simulink model "HybridFEMModel"  (Simulink 7.0)
settings: Solver=FixedStepDiscrete  SolverMode=SingleTasking  StartTime=0.0  StopTime=RunningTime  FixedStep=SampleRate  RelTol=1e-3
undefined symbols (not defined in the file): Alpham, DiscIntNeverNeededParam, Elements, gamma1, gamma2, sample, SampleRate
libraries: simulink x8
(part 2 of 2)

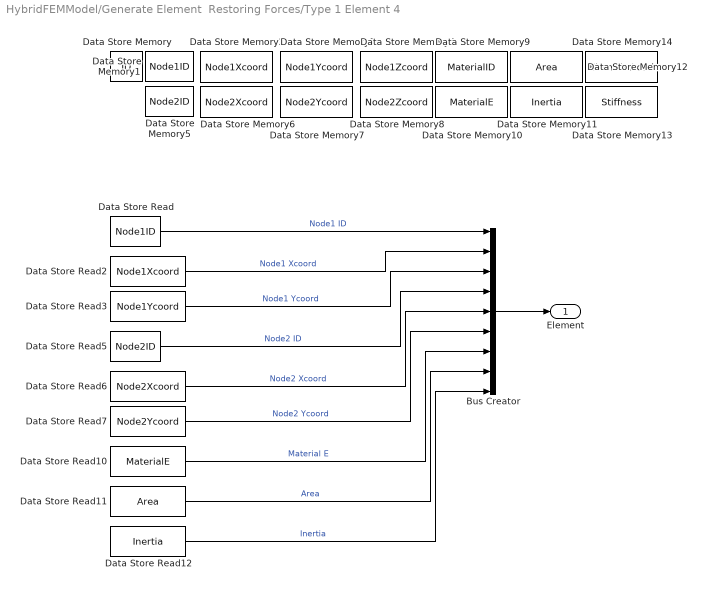
== system HybridFEMModel/Generate Element  Restoring Forces/Type 1 Element 4 ==
  Bus Creator : BusCreator  Inputs=9
  Data Store Memory : DataStoreMemory  DataStoreName=ID  InitialValue=Elements(id).ID  OutDataType=sfix(16)  OutScaling=2^0
  Data Store Memory1 : DataStoreMemory  DataStoreName=Node1ID  InitialValue=Elements(id).Nodes(1).ID  OutDataType=sfix(16)  OutScaling=2^0
  Data Store Memory10 : DataStoreMemory  DataStoreName=MaterialE  InitialValue=Elements(id).Material(1).E  OutDataType=sfix(16)  OutScaling=2^0
  Data Store Memory11 : DataStoreMemory  DataStoreName=Inertia  InitialValue=Elements(id).Inertia  OutDataType=sfix(16)  OutScaling=2^0
  Data Store Memory12 : DataStoreMemory  DataStoreName=Area  InitialValue=Elements(id).Area  OutDataType=sfix(16)  OutScaling=2^0
  Data Store Memory13 : DataStoreMemory  DataStoreName=Stiffness  InitialValue=Elements(id).Stiffness  OutDataType=sfix(16)  OutScaling=2^0
  Data Store Memory14 : DataStoreMemory  DataStoreName=ElemDistLoad  InitialValue=Elements(id).ElemDistLoad  OutDataType=sfix(16)  OutScaling=2^0
  Data Store Memory2 : DataStoreMemory  DataStoreName=Node1Xcoord  InitialValue=Elements(id).Nodes(1).Xcoord  OutDataType=sfix(16)  OutScaling=2^0
  Data Store Memory3 : DataStoreMemory  DataStoreName=Node1Ycoord  InitialValue=Elements(id).Nodes(1).Ycoord  OutDataType=sfix(16)  OutScaling=2^0
  Data Store Memory4 : DataStoreMemory  DataStoreName=Node1Zcoord  InitialValue=Elements(id).Nodes(1).Zcoord  OutDataType=sfix(16)  OutScaling=2^0
  Data Store Memory5 : DataStoreMemory  DataStoreName=Node2ID  InitialValue=Elements(id).Nodes(2).ID  OutDataType=sfix(16)  OutScaling=2^0
  Data Store Memory6 : DataStoreMemory  DataStoreName=Node2Xcoord  InitialValue=Elements(id).Nodes(2).Xcoord  OutDataType=sfix(16)  OutScaling=2^0
  Data Store Memory7 : DataStoreMemory  DataStoreName=Node2Ycoord  InitialValue=Elements(id).Nodes(2).Ycoord  OutDataType=sfix(16)  OutScaling=2^0
  Data Store Memory8 : DataStoreMemory  DataStoreName=Node2Zcoord  InitialValue=Elements(id).Nodes(2).Zcoord  OutDataType=sfix(16)  OutScaling=2^0
  Data Store Memory9 : DataStoreMemory  DataStoreName=MaterialID  InitialValue=Elements(id).Material(1).ID  OutDataType=sfix(16)  OutScaling=2^0
  Data Store Read : DataStoreRead  DataStoreName=Node1ID  SampleTime=-1
  Data Store Read10 : DataStoreRead  DataStoreName=MaterialE  SampleTime=-1
  Data Store Read11 : DataStoreRead  DataStoreName=Area  SampleTime=-1
  Data Store Read12 : DataStoreRead  DataStoreName=Inertia  SampleTime=-1
  Data Store Read2 : DataStoreRead  DataStoreName=Node1Xcoord  SampleTime=-1
  Data Store Read3 : DataStoreRead  DataStoreName=Node1Ycoord  SampleTime=-1
  Data Store Read5 : DataStoreRead  DataStoreName=Node2ID  SampleTime=-1
  Data Store Read6 : DataStoreRead  DataStoreName=Node2Xcoord  SampleTime=-1
  Data Store Read7 : DataStoreRead  DataStoreName=Node2Ycoord  SampleTime=-1
  Element : Outport  OutDataType=sfix(16)  OutScaling=2^0
  wires:
  Bus Creator/1 -> Element/1
  Data Store Read/1 -> Bus Creator/1  "Node1 ID"
  Data Store Read2/1 -> Bus Creator/2  "Node1 Xcoord"
  Data Store Read3/1 -> Bus Creator/3  "Node1 Ycoord"
  Data Store Read5/1 -> Bus Creator/4  "Node2 ID"
  Data Store Read6/1 -> Bus Creator/5  "Node2 Xcoord"
  Data Store Read7/1 -> Bus Creator/6  "Node2 Ycoord"
  Data Store Read10/1 -> Bus Creator/7  "Material E"
  Data Store Read11/1 -> Bus Creator/8  "Area"
  Data Store Read12/1 -> Bus Creator/9  "Inertia"

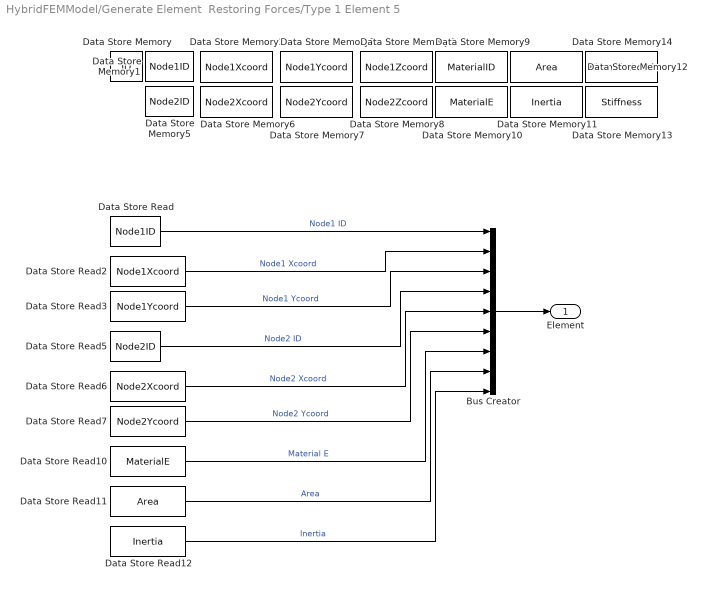
== system HybridFEMModel/Generate Element  Restoring Forces/Type 1 Element 5 ==
  Bus Creator : BusCreator  Inputs=9
  Data Store Memory : DataStoreMemory  DataStoreName=ID  InitialValue=Elements(id).ID  OutDataType=sfix(16)  OutScaling=2^0
  Data Store Memory1 : DataStoreMemory  DataStoreName=Node1ID  InitialValue=Elements(id).Nodes(1).ID  OutDataType=sfix(16)  OutScaling=2^0
  Data Store Memory10 : DataStoreMemory  DataStoreName=MaterialE  InitialValue=Elements(id).Material(1).E  OutDataType=sfix(16)  OutScaling=2^0
  Data Store Memory11 : DataStoreMemory  DataStoreName=Inertia  InitialValue=Elements(id).Inertia  OutDataType=sfix(16)  OutScaling=2^0
  Data Store Memory12 : DataStoreMemory  DataStoreName=Area  InitialValue=Elements(id).Area  OutDataType=sfix(16)  OutScaling=2^0
  Data Store Memory13 : DataStoreMemory  DataStoreName=Stiffness  InitialValue=Elements(id).Stiffness  OutDataType=sfix(16)  OutScaling=2^0
  Data Store Memory14 : DataStoreMemory  DataStoreName=ElemDistLoad  InitialValue=Elements(id).ElemDistLoad  OutDataType=sfix(16)  OutScaling=2^0
  Data Store Memory2 : DataStoreMemory  DataStoreName=Node1Xcoord  InitialValue=Elements(id).Nodes(1).Xcoord  OutDataType=sfix(16)  OutScaling=2^0
  Data Store Memory3 : DataStoreMemory  DataStoreName=Node1Ycoord  InitialValue=Elements(id).Nodes(1).Ycoord  OutDataType=sfix(16)  OutScaling=2^0
  Data Store Memory4 : DataStoreMemory  DataStoreName=Node1Zcoord  InitialValue=Elements(id).Nodes(1).Zcoord  OutDataType=sfix(16)  OutScaling=2^0
  Data Store Memory5 : DataStoreMemory  DataStoreName=Node2ID  InitialValue=Elements(id).Nodes(2).ID  OutDataType=sfix(16)  OutScaling=2^0
  Data Store Memory6 : DataStoreMemory  DataStoreName=Node2Xcoord  InitialValue=Elements(id).Nodes(2).Xcoord  OutDataType=sfix(16)  OutScaling=2^0
  Data Store Memory7 : DataStoreMemory  DataStoreName=Node2Ycoord  InitialValue=Elements(id).Nodes(2).Ycoord  OutDataType=sfix(16)  OutScaling=2^0
  Data Store Memory8 : DataStoreMemory  DataStoreName=Node2Zcoord  InitialValue=Elements(id).Nodes(2).Zcoord  OutDataType=sfix(16)  OutScaling=2^0
  Data Store Memory9 : DataStoreMemory  DataStoreName=MaterialID  InitialValue=Elements(id).Material(1).ID  OutDataType=sfix(16)  OutScaling=2^0
  Data Store Read : DataStoreRead  DataStoreName=Node1ID  SampleTime=-1
  Data Store Read10 : DataStoreRead  DataStoreName=MaterialE  SampleTime=-1
  Data Store Read11 : DataStoreRead  DataStoreName=Area  SampleTime=-1
  Data Store Read12 : DataStoreRead  DataStoreName=Inertia  SampleTime=-1
  Data Store Read2 : DataStoreRead  DataStoreName=Node1Xcoord  SampleTime=-1
  Data Store Read3 : DataStoreRead  DataStoreName=Node1Ycoord  SampleTime=-1
  Data Store Read5 : DataStoreRead  DataStoreName=Node2ID  SampleTime=-1
  Data Store Read6 : DataStoreRead  DataStoreName=Node2Xcoord  SampleTime=-1
  Data Store Read7 : DataStoreRead  DataStoreName=Node2Ycoord  SampleTime=-1
  Element : Outport  OutDataType=sfix(16)  OutScaling=2^0
  wires:
  Data Store Read12/1 -> Bus Creator/9  "Inertia"
  Data Store Read11/1 -> Bus Creator/8  "Area"
  Data Store Read10/1 -> Bus Creator/7  "Material E"
  Data Store Read7/1 -> Bus Creator/6  "Node2 Ycoord"
  Data Store Read6/1 -> Bus Creator/5  "Node2 Xcoord"
  Data Store Read5/1 -> Bus Creator/4  "Node2 ID"
  Data Store Read3/1 -> Bus Creator/3  "Node1 Ycoord"
  Data Store Read2/1 -> Bus Creator/2  "Node1 Xcoord"
  Data Store Read/1 -> Bus Creator/1  "Node1 ID"
  Bus Creator/1 -> Element/1

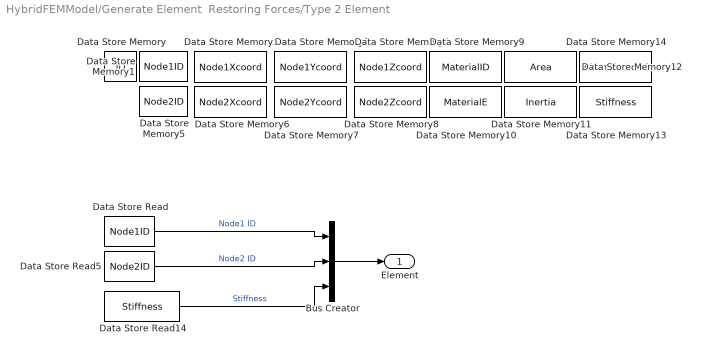
== system HybridFEMModel/Generate Element  Restoring Forces/Type 2 Element ==
  Bus Creator : BusCreator  Inputs=3
  Data Store Memory : DataStoreMemory  DataStoreName=ID  InitialValue=Elements(id).ID  OutDataType=sfix(16)  OutScaling=2^0
  Data Store Memory1 : DataStoreMemory  DataStoreName=Node1ID  InitialValue=Elements(id).Nodes(1).ID  OutDataType=sfix(16)  OutScaling=2^0
  Data Store Memory10 : DataStoreMemory  DataStoreName=MaterialE  InitialValue=Elements(id).Material(1).E  OutDataType=sfix(16)  OutScaling=2^0
  Data Store Memory11 : DataStoreMemory  DataStoreName=Inertia  InitialValue=Elements(id).Inertia  OutDataType=sfix(16)  OutScaling=2^0
  Data Store Memory12 : DataStoreMemory  DataStoreName=Area  InitialValue=Elements(id).Area  OutDataType=sfix(16)  OutScaling=2^0
  Data Store Memory13 : DataStoreMemory  DataStoreName=Stiffness  InitialValue=Elements(id).Stiffness  OutDataType=sfix(16)  OutScaling=2^0
  Data Store Memory14 : DataStoreMemory  DataStoreName=ElemDistLoad  InitialValue=Elements(id).ElemDistLoad  OutDataType=sfix(16)  OutScaling=2^0
  Data Store Memory2 : DataStoreMemory  DataStoreName=Node1Xcoord  InitialValue=Elements(id).Nodes(1).Xcoord  OutDataType=sfix(16)  OutScaling=2^0
  Data Store Memory3 : DataStoreMemory  DataStoreName=Node1Ycoord  InitialValue=Elements(id).Nodes(1).Ycoord  OutDataType=sfix(16)  OutScaling=2^0
  Data Store Memory4 : DataStoreMemory  DataStoreName=Node1Zcoord  InitialValue=Elements(id).Nodes(1).Zcoord  OutDataType=sfix(16)  OutScaling=2^0
  Data Store Memory5 : DataStoreMemory  DataStoreName=Node2ID  InitialValue=Elements(id).Nodes(2).ID  OutDataType=sfix(16)  OutScaling=2^0
  Data Store Memory6 : DataStoreMemory  DataStoreName=Node2Xcoord  InitialValue=Elements(id).Nodes(2).Xcoord  OutDataType=sfix(16)  OutScaling=2^0
  Data Store Memory7 : DataStoreMemory  DataStoreName=Node2Ycoord  InitialValue=Elements(id).Nodes(2).Ycoord  OutDataType=sfix(16)  OutScaling=2^0
  Data Store Memory8 : DataStoreMemory  DataStoreName=Node2Zcoord  InitialValue=Elements(id).Nodes(2).Zcoord  OutDataType=sfix(16)  OutScaling=2^0
  Data Store Memory9 : DataStoreMemory  DataStoreName=MaterialID  InitialValue=Elements(id).Material(1).ID  OutDataType=sfix(16)  OutScaling=2^0
  Data Store Read : DataStoreRead  DataStoreName=Node1ID  SampleTime=-1
  Data Store Read14 : DataStoreRead  DataStoreName=Stiffness  SampleTime=-1
  Data Store Read5 : DataStoreRead  DataStoreName=Node2ID  SampleTime=-1
  Element : Outport  OutDataType=sfix(16)  OutScaling=2^0
  wires:
  Data Store Read14/1 -> Bus Creator/3  "Stiffness"
  Data Store Read5/1 -> Bus Creator/2  "Node2 ID"
  Data Store Read/1 -> Bus Creator/1  "Node1 ID"
  Bus Creator/1 -> Element/1

== system HybridFEMModel/Generate Element  Restoring Forces1/Generate Type 2 Element Restoring Force ==
  Displacement : Inport  OutDataType=sfix(16)  OutScaling=2^0
  Velocity : Inport  Port=2  OutDataType=sfix(16)  OutScaling=2^0
  Element : Inport  Port=3  OutDataType=sfix(16)  OutScaling=2^0
  Timestep : Inport  Port=4  OutDataType=sfix(16)  OutScaling=2^0
  Generate Actuator Command : Stateflow chart
  Act Cmd (m) : Outport  OutDataType=sfix(16)  OutScaling=2^0
  QuadRampCoeffs : Outport  Port=2  OutDataType=sfix(16)  OutScaling=2^0
  wires:
  Generate Actuator Command/1(Command) -> Act Cmd (m)/1
  Displacement/1 -> Generate Actuator Command/2(Displacement)
  Element/1 -> Generate Actuator Command/1(Element)
  Velocity/1 -> Generate Actuator Command/3(Velocity)
  Timestep/1 -> Generate Actuator Command/4(Timestep)
  Generate Actuator Command/2(QuadRampCoeffs) -> QuadRampCoeffs/1

== system HybridFEMModel/Generate Element  Restoring Forces1/Type 2 Element ==
  Bus Creator : BusCreator  Inputs=3
  Data Store Memory : DataStoreMemory  DataStoreName=ID  InitialValue=Elements(id).ID  OutDataType=sfix(16)  OutScaling=2^0
  Data Store Memory1 : DataStoreMemory  DataStoreName=Node1ID  InitialValue=Elements(id).Nodes(1).ID  OutDataType=sfix(16)  OutScaling=2^0
  Data Store Memory10 : DataStoreMemory  DataStoreName=MaterialE  InitialValue=Elements(id).Material(1).E  OutDataType=sfix(16)  OutScaling=2^0
  Data Store Memory11 : DataStoreMemory  DataStoreName=Inertia  InitialValue=Elements(id).Inertia  OutDataType=sfix(16)  OutScaling=2^0
  Data Store Memory12 : DataStoreMemory  DataStoreName=Area  InitialValue=Elements(id).Area  OutDataType=sfix(16)  OutScaling=2^0
  Data Store Memory13 : DataStoreMemory  DataStoreName=Stiffness  InitialValue=Elements(id).Stiffness  OutDataType=sfix(16)  OutScaling=2^0
  Data Store Memory14 : DataStoreMemory  DataStoreName=ElemDistLoad  InitialValue=Elements(id).ElemDistLoad  OutDataType=sfix(16)  OutScaling=2^0
  Data Store Memory2 : DataStoreMemory  DataStoreName=Node1Xcoord  InitialValue=Elements(id).Nodes(1).Xcoord  OutDataType=sfix(16)  OutScaling=2^0
  Data Store Memory3 : DataStoreMemory  DataStoreName=Node1Ycoord  InitialValue=Elements(id).Nodes(1).Ycoord  OutDataType=sfix(16)  OutScaling=2^0
  Data Store Memory4 : DataStoreMemory  DataStoreName=Node1Zcoord  InitialValue=Elements(id).Nodes(1).Zcoord  OutDataType=sfix(16)  OutScaling=2^0
  Data Store Memory5 : DataStoreMemory  DataStoreName=Node2ID  InitialValue=Elements(id).Nodes(2).ID  OutDataType=sfix(16)  OutScaling=2^0
  Data Store Memory6 : DataStoreMemory  DataStoreName=Node2Xcoord  InitialValue=Elements(id).Nodes(2).Xcoord  OutDataType=sfix(16)  OutScaling=2^0
  Data Store Memory7 : DataStoreMemory  DataStoreName=Node2Ycoord  InitialValue=Elements(id).Nodes(2).Ycoord  OutDataType=sfix(16)  OutScaling=2^0
  Data Store Memory8 : DataStoreMemory  DataStoreName=Node2Zcoord  InitialValue=Elements(id).Nodes(2).Zcoord  OutDataType=sfix(16)  OutScaling=2^0
  Data Store Memory9 : DataStoreMemory  DataStoreName=MaterialID  InitialValue=Elements(id).Material(1).ID  OutDataType=sfix(16)  OutScaling=2^0
  Data Store Read : DataStoreRead  DataStoreName=Node1ID  SampleTime=-1
  Data Store Read14 : DataStoreRead  DataStoreName=Stiffness  SampleTime=-1
  Data Store Read5 : DataStoreRead  DataStoreName=Node2ID  SampleTime=-1
  Element : Outport  OutDataType=sfix(16)  OutScaling=2^0
  wires:
  Data Store Read14/1 -> Bus Creator/3  "Stiffness"
  Data Store Read5/1 -> Bus Creator/2  "Node2 ID"
  Data Store Read/1 -> Bus Creator/1  "Node1 ID"
  Bus Creator/1 -> Element/1

== system HybridFEMModel/Linear AIC/Tracking Indicator ==
  note: TI
  note: TA
  note: A
  note: dm
  note: dc
  In1 : Inport  OutDataType=sfix(16)  OutScaling=2^0
  In2 : Inport  Port=2  OutDataType=sfix(16)  OutScaling=2^0
  A : Subsystem
  Gain : Gain  Gain=0.5  ParameterDataType=sfix(16)  ParameterScaling=2^0  OutDataType=sfix(16)  OutScaling=2^0
  Scope : Scope
      settings: SaveName=ScopeData4
  Sum : Sum  Inputs=|+-  OutDataType=sfix(16)  OutScaling=2^0
  TA : Subsystem
  Out1 : Outport  OutDataType=sfix(16)  OutScaling=2^0
  wires:
  Gain/1 -> Scope/1, Out1/1
  Sum/1 -> Gain/1
  A/1(Out1) -> Sum/1
  TA/1(Out1) -> Sum/2
  In1/1 -> TA/1(In1), A/1(In1)
  In2/1 -> TA/2(In2), A/2(In2)

== system HybridFEMModel/Linear AIC/adaptive block ==
  indicator : Inport  OutDataType=sfix(16)  OutScaling=2^0
  Discrete-Time Integrator : DiscreteIntegrator  SampleTime=sample  OutDataType=sfix(16)  OutScaling=2^0  ICPrevOutput=DiscIntNeverNeededParam  ICPrevScaledInput=DiscIntNeverNeededParam
  Gain : Gain  ParameterDataType=sfix(16)  ParameterScaling=2^0  OutDataType=sfix(16)  OutScaling=2^0
  Product : Product  OutDataType=sfix(16)  OutScaling=2^0  RndMeth=Zero
  Product1 : Product  OutDataType=sfix(16)  OutScaling=2^0  RndMeth=Zero
  Sum : Sum  Inputs=|++  OutDataType=sfix(16)  OutScaling=2^0
  gamma1 : Constant  Value=gamma1  OutDataType=sfix(16)  OutScaling=2^0
  gamma2 : Constant  Value=gamma2  OutDataType=sfix(16)  OutScaling=2^0
  Out1 : Outport  OutDataType=sfix(16)  OutScaling=2^0
  wires:
  Gain/1 -> Product1/1, Discrete-Time Integrator/1
  Product1/1 -> Sum/2
  indicator/1 -> Gain/1
  Sum/1 -> Out1/1
  Product/1 -> Sum/1
  gamma1/1 -> Product1/2
  gamma2/1 -> Product/2
  Discrete-Time Integrator/1 -> Product/1

== system HybridFEMModel/Linear AIC/inverse compensator ==
  note: dc
  note: d(alpha)
  note: dp
  In1 : Inport  OutDataType=sfix(16)  OutScaling=2^0
  In2 : Inport  Port=2  OutDataType=sfix(16)  OutScaling=2^0
  Discrete Transfer Fcn : DiscreteTransferFcn  Numerator=[1 -1]  Denominator=[1 0]  SampleTime=sample
  Product : Product  OutDataType=sfix(16)  OutScaling=2^0  RndMeth=Zero
  Scope : Scope
  Sum2 : Sum  Inputs=|++  OutDataType=sfix(16)  OutScaling=2^0
  Sum5 : Sum  Inputs=|++  OutDataType=sfix(16)  OutScaling=2^0
  Unit Delay : UnitDelay  SampleTime=sample
  alpham : Constant  Value=Alpham  OutDataType=sfix(16)  OutScaling=2^0
  Out1 : Outport  OutDataType=sfix(16)  OutScaling=2^0
  wires:
  In1/1 -> Discrete Transfer Fcn/1, Unit Delay/1
  In2/1 -> Sum5/1
  alpham/1 -> Sum5/2
  Discrete Transfer Fcn/1 -> Product/1
  Sum5/1 -> Product/2, Scope/1
  Unit Delay/1 -> Sum2/1
  Product/1 -> Sum2/2
  Sum2/1 -> Out1/1

== system HybridFEMModel/Linear AIC1/Tracking Indicator ==
  note: dc
  note: dm
  note: A
  note: TA
  note: TI
  In1 : Inport  OutDataType=sfix(16)  OutScaling=2^0
  In2 : Inport  Port=2  OutDataType=sfix(16)  OutScaling=2^0
  A : Subsystem
  Gain : Gain  Gain=0.5  ParameterDataType=sfix(16)  ParameterScaling=2^0  OutDataType=sfix(16)  OutScaling=2^0
  Scope : Scope
      settings: SaveName=ScopeData4
  Sum : Sum  Inputs=|+-  OutDataType=sfix(16)  OutScaling=2^0
  TA : Subsystem
  Out1 : Outport  OutDataType=sfix(16)  OutScaling=2^0
  wires:
  In2/1 -> A/2(In2), TA/2(In2)
  In1/1 -> A/1(In1), TA/1(In1)
  TA/1(Out1) -> Sum/2
  A/1(Out1) -> Sum/1
  Sum/1 -> Gain/1
  Gain/1 -> Out1/1, Scope/1

== system HybridFEMModel/Linear AIC1/adaptive block ==
  indicator : Inport  OutDataType=sfix(16)  OutScaling=2^0
  Discrete-Time Integrator : DiscreteIntegrator  SampleTime=sample  OutDataType=sfix(16)  OutScaling=2^0  ICPrevOutput=DiscIntNeverNeededParam  ICPrevScaledInput=DiscIntNeverNeededParam
  Gain : Gain  ParameterDataType=sfix(16)  ParameterScaling=2^0  OutDataType=sfix(16)  OutScaling=2^0
  Product : Product  OutDataType=sfix(16)  OutScaling=2^0  RndMeth=Zero
  Product1 : Product  OutDataType=sfix(16)  OutScaling=2^0  RndMeth=Zero
  Sum : Sum  Inputs=|++  OutDataType=sfix(16)  OutScaling=2^0
  gamma1 : Constant  Value=gamma1  OutDataType=sfix(16)  OutScaling=2^0
  gamma2 : Constant  Value=gamma2  OutDataType=sfix(16)  OutScaling=2^0
  Out1 : Outport  OutDataType=sfix(16)  OutScaling=2^0
  wires:
  Discrete-Time Integrator/1 -> Product/1
  gamma2/1 -> Product/2
  gamma1/1 -> Product1/2
  Product/1 -> Sum/1
  Sum/1 -> Out1/1
  indicator/1 -> Gain/1
  Product1/1 -> Sum/2
  Gain/1 -> Discrete-Time Integrator/1, Product1/1

== system HybridFEMModel/Linear AIC1/inverse compensator ==
  note: dp
  note: d(alpha)
  note: dc
  In1 : Inport  OutDataType=sfix(16)  OutScaling=2^0
  In2 : Inport  Port=2  OutDataType=sfix(16)  OutScaling=2^0
  Discrete Transfer Fcn : DiscreteTransferFcn  Numerator=[1 -1]  Denominator=[1 0]  SampleTime=sample
  Product : Product  OutDataType=sfix(16)  OutScaling=2^0  RndMeth=Zero
  Scope : Scope
  Sum2 : Sum  Inputs=|++  OutDataType=sfix(16)  OutScaling=2^0
  Sum5 : Sum  Inputs=|++  OutDataType=sfix(16)  OutScaling=2^0
  Unit Delay : UnitDelay  SampleTime=sample
  alpham : Constant  Value=Alpham  OutDataType=sfix(16)  OutScaling=2^0
  Out1 : Outport  OutDataType=sfix(16)  OutScaling=2^0
  wires:
  Sum2/1 -> Out1/1
  Product/1 -> Sum2/2
  Unit Delay/1 -> Sum2/1
  Sum5/1 -> Scope/1, Product/2
  Discrete Transfer Fcn/1 -> Product/1
  alpham/1 -> Sum5/2
  In2/1 -> Sum5/1
  In1/1 -> Unit Delay/1, Discrete Transfer Fcn/1

== system HybridFEMModel/Quad Ramp Gen AIC/Tracking Indicator ==
  note: dc
  note: dm
  note: A
  note: TA
  note: TI
  In1 : Inport  OutDataType=sfix(16)  OutScaling=2^0
  In2 : Inport  Port=2  OutDataType=sfix(16)  OutScaling=2^0
  A : Subsystem
  Gain : Gain  Gain=0.5  ParameterDataType=sfix(16)  ParameterScaling=2^0  OutDataType=sfix(16)  OutScaling=2^0
  Scope : Scope
      settings: SaveName=ScopeData4
  Sum : Sum  Inputs=|+-  OutDataType=sfix(16)  OutScaling=2^0
  TA : Subsystem
  Out1 : Outport  OutDataType=sfix(16)  OutScaling=2^0
  wires:
  In2/1 -> A/2(In2), TA/2(In2)
  In1/1 -> A/1(In1), TA/1(In1)
  TA/1(Out1) -> Sum/2
  A/1(Out1) -> Sum/1
  Sum/1 -> Gain/1
  Gain/1 -> Out1/1, Scope/1

== system HybridFEMModel/Quad Ramp Gen AIC/adaptive block ==
  indicator : Inport  OutDataType=sfix(16)  OutScaling=2^0
  Discrete-Time Integrator : DiscreteIntegrator  SampleTime=sample  OutDataType=sfix(16)  OutScaling=2^0  ICPrevOutput=DiscIntNeverNeededParam  ICPrevScaledInput=DiscIntNeverNeededParam
  Gain : Gain  ParameterDataType=sfix(16)  ParameterScaling=2^0  OutDataType=sfix(16)  OutScaling=2^0
  Product : Product  OutDataType=sfix(16)  OutScaling=2^0  RndMeth=Zero
  Product1 : Product  OutDataType=sfix(16)  OutScaling=2^0  RndMeth=Zero
  Sum : Sum  Inputs=|++  OutDataType=sfix(16)  OutScaling=2^0
  gamma1 : Constant  Value=gamma1  OutDataType=sfix(16)  OutScaling=2^0
  gamma2 : Constant  Value=gamma2  OutDataType=sfix(16)  OutScaling=2^0
  Out1 : Outport  OutDataType=sfix(16)  OutScaling=2^0
  wires:
  Discrete-Time Integrator/1 -> Product/1
  gamma2/1 -> Product/2
  gamma1/1 -> Product1/2
  Product/1 -> Sum/1
  Sum/1 -> Out1/1
  indicator/1 -> Gain/1
  Product1/1 -> Sum/2
  Gain/1 -> Discrete-Time Integrator/1, Product1/1

== system HybridFEMModel/Quad Ramp Gen AIC/inverse compensator ==
  note: dp
  note: d(alpha)
  note: dc
  In1 : Inport  OutDataType=sfix(16)  OutScaling=2^0
  In2 : Inport  Port=2  OutDataType=sfix(16)  OutScaling=2^0
  Discrete Transfer Fcn : DiscreteTransferFcn  Numerator=[1 -1]  Denominator=[1 0]  SampleTime=sample
  Product : Product  OutDataType=sfix(16)  OutScaling=2^0  RndMeth=Zero
  Scope : Scope
  Sum2 : Sum  Inputs=|++  OutDataType=sfix(16)  OutScaling=2^0
  Sum5 : Sum  Inputs=|++  OutDataType=sfix(16)  OutScaling=2^0
  Unit Delay : UnitDelay  SampleTime=sample
  alpham : Constant  Value=Alpham  OutDataType=sfix(16)  OutScaling=2^0
  Out1 : Outport  OutDataType=sfix(16)  OutScaling=2^0
  wires:
  Sum2/1 -> Out1/1
  Product/1 -> Sum2/2
  Unit Delay/1 -> Sum2/1
  Sum5/1 -> Scope/1, Product/2
  Discrete Transfer Fcn/1 -> Product/1
  alpham/1 -> Sum5/2
  In2/1 -> Sum5/1
  In1/1 -> Unit Delay/1, Discrete Transfer Fcn/1

== system HybridFEMModel/Linear AIC/Tracking Indicator/A ==
  note: TI
  note: dm
  note: dc
  In1 : Inport  OutDataType=sfix(16)  OutScaling=2^0
  In2 : Inport  Port=2  OutDataType=sfix(16)  OutScaling=2^0
  Gain : Gain  Gain=0.5  ParameterDataType=sfix(16)  ParameterScaling=2^0  OutDataType=sfix(16)  OutScaling=2^0
  Product1 : Product  OutDataType=sfix(16)  OutScaling=2^0  RndMeth=Zero
  Sum2 : Sum  Inputs=|++  OutDataType=sfix(16)  OutScaling=2^0
  Sum3 : Sum  Inputs=|+-  OutDataType=sfix(16)  OutScaling=2^0
  Unit Delay : UnitDelay  SampleTime=sample
  Unit Delay1 : UnitDelay  SampleTime=sample
  accumulation : DiscreteTransferFcn  Numerator=[1 0]  Denominator=[1 -1]  SampleTime=sample
  Out1 : Outport  OutDataType=sfix(16)  OutScaling=2^0
  wires:
  accumulation/1 -> Out1/1
  Gain/1 -> accumulation/1
  Product1/1 -> Gain/1
  Sum3/1 -> Product1/2
  Sum2/1 -> Product1/1
  Unit Delay1/1 -> Sum3/2
  Unit Delay/1 -> Sum2/1
  In2/1 -> Unit Delay1/1, Sum3/1
  In1/1 -> Sum2/2, Unit Delay/1

== system HybridFEMModel/Linear AIC/Tracking Indicator/TA ==
  note: TI
  note: dc
  note: dm
  In1 : Inport  OutDataType=sfix(16)  OutScaling=2^0
  In2 : Inport  Port=2  OutDataType=sfix(16)  OutScaling=2^0
  Gain : Gain  Gain=0.5  ParameterDataType=sfix(16)  ParameterScaling=2^0  OutDataType=sfix(16)  OutScaling=2^0
  Product1 : Product  OutDataType=sfix(16)  OutScaling=2^0  RndMeth=Zero
  Sum2 : Sum  Inputs=|++  OutDataType=sfix(16)  OutScaling=2^0
  Sum3 : Sum  Inputs=|+-  OutDataType=sfix(16)  OutScaling=2^0
  Unit Delay : UnitDelay  SampleTime=sample
  Unit Delay1 : UnitDelay  SampleTime=sample
  accumulation : DiscreteTransferFcn  Numerator=[1 0]  Denominator=[1 -1]  SampleTime=sample
  Out1 : Outport  OutDataType=sfix(16)  OutScaling=2^0
  wires:
  accumulation/1 -> Out1/1
  Gain/1 -> accumulation/1
  Product1/1 -> Gain/1
  Sum3/1 -> Product1/2
  Sum2/1 -> Product1/1
  Unit Delay1/1 -> Sum3/2
  Unit Delay/1 -> Sum2/1
  In1/1 -> Unit Delay1/1, Sum3/1
  In2/1 -> Sum2/2, Unit Delay/1

== system HybridFEMModel/Linear AIC1/Tracking Indicator/A ==
  note: dc
  note: dm
  note: TI
  In1 : Inport  OutDataType=sfix(16)  OutScaling=2^0
  In2 : Inport  Port=2  OutDataType=sfix(16)  OutScaling=2^0
  Gain : Gain  Gain=0.5  ParameterDataType=sfix(16)  ParameterScaling=2^0  OutDataType=sfix(16)  OutScaling=2^0
  Product1 : Product  OutDataType=sfix(16)  OutScaling=2^0  RndMeth=Zero
  Sum2 : Sum  Inputs=|++  OutDataType=sfix(16)  OutScaling=2^0
  Sum3 : Sum  Inputs=|+-  OutDataType=sfix(16)  OutScaling=2^0
  Unit Delay : UnitDelay  SampleTime=sample
  Unit Delay1 : UnitDelay  SampleTime=sample
  accumulation : DiscreteTransferFcn  Numerator=[1 0]  Denominator=[1 -1]  SampleTime=sample
  Out1 : Outport  OutDataType=sfix(16)  OutScaling=2^0
  wires:
  In1/1 -> Unit Delay/1, Sum2/2
  In2/1 -> Sum3/1, Unit Delay1/1
  Unit Delay/1 -> Sum2/1
  Unit Delay1/1 -> Sum3/2
  Sum2/1 -> Product1/1
  Sum3/1 -> Product1/2
  Product1/1 -> Gain/1
  Gain/1 -> accumulation/1
  accumulation/1 -> Out1/1

== system HybridFEMModel/Linear AIC1/Tracking Indicator/TA ==
  note: dm
  note: dc
  note: TI
  In1 : Inport  OutDataType=sfix(16)  OutScaling=2^0
  In2 : Inport  Port=2  OutDataType=sfix(16)  OutScaling=2^0
  Gain : Gain  Gain=0.5  ParameterDataType=sfix(16)  ParameterScaling=2^0  OutDataType=sfix(16)  OutScaling=2^0
  Product1 : Product  OutDataType=sfix(16)  OutScaling=2^0  RndMeth=Zero
  Sum2 : Sum  Inputs=|++  OutDataType=sfix(16)  OutScaling=2^0
  Sum3 : Sum  Inputs=|+-  OutDataType=sfix(16)  OutScaling=2^0
  Unit Delay : UnitDelay  SampleTime=sample
  Unit Delay1 : UnitDelay  SampleTime=sample
  accumulation : DiscreteTransferFcn  Numerator=[1 0]  Denominator=[1 -1]  SampleTime=sample
  Out1 : Outport  OutDataType=sfix(16)  OutScaling=2^0
  wires:
  In2/1 -> Unit Delay/1, Sum2/2
  In1/1 -> Sum3/1, Unit Delay1/1
  Unit Delay/1 -> Sum2/1
  Unit Delay1/1 -> Sum3/2
  Sum2/1 -> Product1/1
  Sum3/1 -> Product1/2
  Product1/1 -> Gain/1
  Gain/1 -> accumulation/1
  accumulation/1 -> Out1/1

== system HybridFEMModel/Quad Ramp Gen AIC/Tracking Indicator/A ==
  note: dc
  note: dm
  note: TI
  In1 : Inport  OutDataType=sfix(16)  OutScaling=2^0
  In2 : Inport  Port=2  OutDataType=sfix(16)  OutScaling=2^0
  Gain : Gain  Gain=0.5  ParameterDataType=sfix(16)  ParameterScaling=2^0  OutDataType=sfix(16)  OutScaling=2^0
  Product1 : Product  OutDataType=sfix(16)  OutScaling=2^0  RndMeth=Zero
  Sum2 : Sum  Inputs=|++  OutDataType=sfix(16)  OutScaling=2^0
  Sum3 : Sum  Inputs=|+-  OutDataType=sfix(16)  OutScaling=2^0
  Unit Delay : UnitDelay  SampleTime=sample
  Unit Delay1 : UnitDelay  SampleTime=sample
  accumulation : DiscreteTransferFcn  Numerator=[1 0]  Denominator=[1 -1]  SampleTime=sample
  Out1 : Outport  OutDataType=sfix(16)  OutScaling=2^0
  wires:
  In1/1 -> Unit Delay/1, Sum2/2
  In2/1 -> Sum3/1, Unit Delay1/1
  Unit Delay/1 -> Sum2/1
  Unit Delay1/1 -> Sum3/2
  Sum2/1 -> Product1/1
  Sum3/1 -> Product1/2
  Product1/1 -> Gain/1
  Gain/1 -> accumulation/1
  accumulation/1 -> Out1/1

== system HybridFEMModel/Quad Ramp Gen AIC/Tracking Indicator/TA ==
  note: dm
  note: dc
  note: TI
  In1 : Inport  OutDataType=sfix(16)  OutScaling=2^0
  In2 : Inport  Port=2  OutDataType=sfix(16)  OutScaling=2^0
  Gain : Gain  Gain=0.5  ParameterDataType=sfix(16)  ParameterScaling=2^0  OutDataType=sfix(16)  OutScaling=2^0
  Product1 : Product  OutDataType=sfix(16)  OutScaling=2^0  RndMeth=Zero
  Sum2 : Sum  Inputs=|++  OutDataType=sfix(16)  OutScaling=2^0
  Sum3 : Sum  Inputs=|+-  OutDataType=sfix(16)  OutScaling=2^0
  Unit Delay : UnitDelay  SampleTime=sample
  Unit Delay1 : UnitDelay  SampleTime=sample
  accumulation : DiscreteTransferFcn  Numerator=[1 0]  Denominator=[1 -1]  SampleTime=sample
  Out1 : Outport  OutDataType=sfix(16)  OutScaling=2^0
  wires:
  In2/1 -> Unit Delay/1, Sum2/2
  In1/1 -> Sum3/1, Unit Delay1/1
  Unit Delay/1 -> Sum2/1
  Unit Delay1/1 -> Sum3/2
  Sum2/1 -> Product1/1
  Sum3/1 -> Product1/2
  Product1/1 -> Gain/1
  Gain/1 -> accumulation/1
  accumulation/1 -> Out1/1

== matlab function Generate Element Restoring Forces/Generate Type 2 Element Restoring Force/Type 2 Element RF ==
  data: Nodes output inherited; Element input inherited; RF output inherited; NumFreeDOF input inherited; Displacement input inherited; ActuatorRF input inherited
% get restoring force for the element
% returns (6x1) restoring force vector of element in global coordinates
function [Nodes,RF] = fcn(Element, NumFreeDOF, Displacement, ActuatorRF)

%% Simulation flag
simulation = 1;

%% Input mapping
Node1ID = Element(1);
Node2ID = Element(2);
Stiffness = Element(3);
Nodes = [Node1ID,Node2ID];

% Get distance between nodes
I1 = Node1ID;
I2 = Node2ID;

% preset arrays
SE = zeros(6,6);
    
% Form Stiffness Matrix
SE(1, 1) = Stiffness;
SE(1, 4) = -Stiffness;
SE(4, 4) = Stiffness;
SE(4, 1) = SE(1,4);

% Check if it is a simulation or using real RF
if (simulation == 1)
    %create the displacement Ue (6x1) vector of the element in global coordinates
    Ue = zeros(6, 1);
    if (I1 * 3) <= NumFreeDOF
        Ue(1, 1) = Displacement(I1 * 3 - 2, 1);
        Ue(2, 1) = Displacement(I1 * 3 - 1, 1);
        Ue(3, 1) = Displacement(I1 * 3, 1);
    end
    if (I2 * 3) <= NumFreeDOF
        Ue(4, 1) = Displacement(I2 * 3 - 2, 1);
        Ue(5, 1) = Displacement(I2 * 3 - 1, 1);
        Ue(6, 1) = Displacement(I2 * 3, 1);
    end
    RF = SE*Ue;  %resisting (6x1) resisting force vector of element in global coordinates
else
    RestoringForce = zeros(6,1);
    RestoringForce(1,1) = -ActuatorRF;
    RestoringForce(4,1) = ActuatorRF;
	RF = RestoringForce;
end

== matlab function Generate Element Restoring Forces/Form Total Restoring Force Vector/Form Restoring Force Vector ==
  data: Nodes_muxed input inherited; RF_muxed input inherited; TotalRF output inherited
function TotalRF = eml(Nodes_muxed,RF_muxed)
% This block supports the Embedded MATLAB subset.
% See the help menu for details. 

NumFreeDOF = 12;
TotalRF = zeros(NumFreeDOF,1);

for i = 2:2:length(Nodes_muxed)
    N1 = Nodes_muxed(i-1);
    N2 = Nodes_muxed(i);
    if (3 * N1) <= NumFreeDOF
        TotalRF(N1 * 3 - 2, 1) = RF_muxed(1+(6*(i-2)/2)) + TotalRF(N1 * 3 - 2, 1);
        TotalRF(N1 * 3 - 1, 1) = RF_muxed(2+(6*(i-2)/2)) + TotalRF(N1 * 3 - 1, 1);
        TotalRF(N1 * 3, 1) = RF_muxed(3+(6*(i-2)/2)) + TotalRF(N1 * 3, 1);
    end
    if (3 * N2) <= NumFreeDOF
        TotalRF(N2 * 3 - 2, 1) = RF_muxed(4+(6*(i-2)/2)) + TotalRF(N2 * 3 - 2, 1);
        TotalRF(N2 * 3 - 1, 1) = RF_muxed(5+(6*(i-2)/2)) + TotalRF(N2 * 3 - 1, 1);
        TotalRF(N2 * 3, 1) = RF_muxed(6+(6*(i-2)/2)) + TotalRF(N2 * 3, 1);
    end
end

== matlab function Generate Element Restoring Forces/Generate Type 1 Element Restoring Force/Type 1 Element RF ==
  data: Nodes output inherited; Element input inherited; RF output inherited; NumFreeDOF input inherited; Displacement input inherited
% get restoring force for the element
% returns (6x1) restoring force vector of element in global coordinates
function [Nodes,RF] = eml(Element, NumFreeDOF, Displacement)

%% Input mapping
Node1ID = Element(1);
Node1Xcoord = Element(2);
Node1Ycoord = Element(3);
Node2ID = Element(4);
Node2Xcoord = Element(5);
Node2Ycoord = Element(6);
MaterialE = Element(7);
Area = Element(8);
Inertia = Element(9);
Nodes = [Node1ID,Node2ID];

% Get distance between nodes
I1 = Node1ID;
I2 = Node2ID;
X21 = Node2Xcoord - Node1Xcoord;
Y21 = Node2Ycoord - Node1Ycoord;
EL = sqrt(X21 * X21 + Y21 * Y21);
EAL = MaterialE * Area / EL;
EIZL = MaterialE * Inertia / EL;
%calculation of density (the uniform load is only taken into account)
SEP = zeros(6);
SEP(1, 1) = EAL;
SEP(1, 4) = -EAL;
SEP(4, 4) = EAL;
SEP(2, 2) = 12 * EIZL / EL ^ 2;
SEP(2, 3) = 6 * EIZL / EL;
SEP(2, 5) = -SEP(2, 2);
SEP(2, 6) = SEP(2, 3);
SEP(3, 3) = 4 * EIZL;
SEP(3, 5) = -6 * EIZL / EL;
SEP(3, 6) = 2 * EIZL;
SEP(5, 5) = 12 * EIZL / EL ^ 2;
SEP(5, 6) = -6 * EIZL / EL;
SEP(6, 6) = 4 * EIZL;
for i = 1:6
   for j = i:6
      SEP(j, i) = SEP(i, j);
   end
end
DCOS = zeros(3,3);
DCOS(1, 1) = X21 / EL;
DCOS(1, 2) = Y21 / EL;
DCOS(1, 3) = 0;
DCOS(2, 1) = -DCOS(1, 2);
DCOS(2, 2) = DCOS(1, 1);
DCOS(2, 3) = 0;
DCOS(3, 1) = 0;
DCOS(3, 2) = 0;
DCOS(3, 3) = 1;
ALMBDA = zeros(6);       
for i = 1:2
   IK = 3 * (i - 1);
   for j = 1:3
      for k = 1:3
         ALMBDA(j + IK, k + IK) = DCOS(j, k);
      end
   end
end
SE = SEP * ALMBDA;
SEP = SE;
SE = ALMBDA' * SEP;
%create the displacement Ue (6x1) vector of the element in global coordinates
Ue = zeros(6,1);
if (I1 * 3) <= NumFreeDOF
    Ue(1, 1) = Displacement(I1 * 3 - 2, 1);
    Ue(2, 1) = Displacement(I1 * 3 - 1, 1);
    Ue(3, 1) = Displacement(I1 * 3, 1);
end
if (I2 * 3) <= NumFreeDOF
    Ue(4, 1) = Displacement(I2 * 3 - 2, 1);
    Ue(5, 1) = Displacement(I2 * 3 - 1, 1);
    Ue(6, 1) = Displacement(I2 * 3, 1);
end
RF = SE * Ue;  %resisting (6x1) resisting force vector of element in global coordinates

== matlab function Generate Element Restoring Forces/Generate Type 1 Element Restoring Force1/Type 1 Element RF ==
  data: Nodes output inherited; Element input inherited; RF output inherited; NumFreeDOF input inherited; Displacement input inherited
% get restoring force for the element
% returns (6x1) restoring force vector of element in global coordinates
function [Nodes,RF] = eml(Element, NumFreeDOF, Displacement)

%% Input mapping
Node1ID = Element(1);
Node1Xcoord = Element(2);
Node1Ycoord = Element(3);
Node2ID = Element(4);
Node2Xcoord = Element(5);
Node2Ycoord = Element(6);
MaterialE = Element(7);
Area = Element(8);
Inertia = Element(9);
Nodes = [Node1ID,Node2ID];

% Get distance between nodes
I1 = Node1ID;
I2 = Node2ID;
X21 = Node2Xcoord - Node1Xcoord;
Y21 = Node2Ycoord - Node1Ycoord;
EL = sqrt(X21 * X21 + Y21 * Y21);
EAL = MaterialE * Area / EL;
EIZL = MaterialE * Inertia / EL;
%calculation of density (the uniform load is only taken into account)
SEP = zeros(6);
SEP(1, 1) = EAL;
SEP(1, 4) = -EAL;
SEP(4, 4) = EAL;
SEP(2, 2) = 12 * EIZL / EL ^ 2;
SEP(2, 3) = 6 * EIZL / EL;
SEP(2, 5) = -SEP(2, 2);
SEP(2, 6) = SEP(2, 3);
SEP(3, 3) = 4 * EIZL;
SEP(3, 5) = -6 * EIZL / EL;
SEP(3, 6) = 2 * EIZL;
SEP(5, 5) = 12 * EIZL / EL ^ 2;
SEP(5, 6) = -6 * EIZL / EL;
SEP(6, 6) = 4 * EIZL;
for i = 1:6
   for j = i:6
      SEP(j, i) = SEP(i, j);
   end
end
DCOS = zeros(3,3);
DCOS(1, 1) = X21 / EL;
DCOS(1, 2) = Y21 / EL;
DCOS(1, 3) = 0;
DCOS(2, 1) = -DCOS(1, 2);
DCOS(2, 2) = DCOS(1, 1);
DCOS(2, 3) = 0;
DCOS(3, 1) = 0;
DCOS(3, 2) = 0;
DCOS(3, 3) = 1;
ALMBDA = zeros(6);       
for i = 1:2
   IK = 3 * (i - 1);
   for j = 1:3
      for k = 1:3
         ALMBDA(j + IK, k + IK) = DCOS(j, k);
      end
   end
end
SE = SEP * ALMBDA;
SEP = SE;
SE = ALMBDA' * SEP;
%create the displacement Ue (6x1) vector of the element in global coordinates
Ue = zeros(6,1);
if (I1 * 3) <= NumFreeDOF
    Ue(1, 1) = Displacement(I1 * 3 - 2, 1);
    Ue(2, 1) = Displacement(I1 * 3 - 1, 1);
    Ue(3, 1) = Displacement(I1 * 3, 1);
end
if (I2 * 3) <= NumFreeDOF
    Ue(4, 1) = Displacement(I2 * 3 - 2, 1);
    Ue(5, 1) = Displacement(I2 * 3 - 1, 1);
    Ue(6, 1) = Displacement(I2 * 3, 1);
end
RF = SE * Ue;  %resisting (6x1) resisting force vector of element in global coordinates

== matlab function Generate Element Restoring Forces/Generate Type 1 Element Restoring Force2/Type 1 Element RF ==
  data: Nodes output inherited; Element input inherited; RF output inherited; NumFreeDOF input inherited; Displacement input inherited
% get restoring force for the element
% returns (6x1) restoring force vector of element in global coordinates
function [Nodes,RF] = eml(Element, NumFreeDOF, Displacement)

%% Input mapping
Node1ID = Element(1);
Node1Xcoord = Element(2);
Node1Ycoord = Element(3);
Node2ID = Element(4);
Node2Xcoord = Element(5);
Node2Ycoord = Element(6);
MaterialE = Element(7);
Area = Element(8);
Inertia = Element(9);
Nodes = [Node1ID,Node2ID];

% Get distance between nodes
I1 = Node1ID;
I2 = Node2ID;
X21 = Node2Xcoord - Node1Xcoord;
Y21 = Node2Ycoord - Node1Ycoord;
EL = sqrt(X21 * X21 + Y21 * Y21);
EAL = MaterialE * Area / EL;
EIZL = MaterialE * Inertia / EL;
%calculation of density (the uniform load is only taken into account)
SEP = zeros(6);
SEP(1, 1) = EAL;
SEP(1, 4) = -EAL;
SEP(4, 4) = EAL;
SEP(2, 2) = 12 * EIZL / EL ^ 2;
SEP(2, 3) = 6 * EIZL / EL;
SEP(2, 5) = -SEP(2, 2);
SEP(2, 6) = SEP(2, 3);
SEP(3, 3) = 4 * EIZL;
SEP(3, 5) = -6 * EIZL / EL;
SEP(3, 6) = 2 * EIZL;
SEP(5, 5) = 12 * EIZL / EL ^ 2;
SEP(5, 6) = -6 * EIZL / EL;
SEP(6, 6) = 4 * EIZL;
for i = 1:6
   for j = i:6
      SEP(j, i) = SEP(i, j);
   end
end
DCOS = zeros(3,3);
DCOS(1, 1) = X21 / EL;
DCOS(1, 2) = Y21 / EL;
DCOS(1, 3) = 0;
DCOS(2, 1) = -DCOS(1, 2);
DCOS(2, 2) = DCOS(1, 1);
DCOS(2, 3) = 0;
DCOS(3, 1) = 0;
DCOS(3, 2) = 0;
DCOS(3, 3) = 1;
ALMBDA = zeros(6);       
for i = 1:2
   IK = 3 * (i - 1);
   for j = 1:3
      for k = 1:3
         ALMBDA(j + IK, k + IK) = DCOS(j, k);
      end
   end
end
SE = SEP * ALMBDA;
SEP = SE;
SE = ALMBDA' * SEP;
%create the displacement Ue (6x1) vector of the element in global coordinates
Ue = zeros(6,1);
if (I1 * 3) <= NumFreeDOF
    Ue(1, 1) = Displacement(I1 * 3 - 2, 1);
    Ue(2, 1) = Displacement(I1 * 3 - 1, 1);
    Ue(3, 1) = Displacement(I1 * 3, 1);
end
if (I2 * 3) <= NumFreeDOF
    Ue(4, 1) = Displacement(I2 * 3 - 2, 1);
    Ue(5, 1) = Displacement(I2 * 3 - 1, 1);
    Ue(6, 1) = Displacement(I2 * 3, 1);
end
RF = SE * Ue;  %resisting (6x1) resisting force vector of element in global coordinates

== matlab function Generate Element Restoring Forces/Generate Type 1 Element Restoring Force3/Type 1 Element RF ==
  data: Nodes output inherited; Element input inherited; RF output inherited; NumFreeDOF input inherited; Displacement input inherited
% get restoring force for the element
% returns (6x1) restoring force vector of element in global coordinates
function [Nodes,RF] = eml(Element, NumFreeDOF, Displacement)

%% Input mapping
Node1ID = Element(1);
Node1Xcoord = Element(2);
Node1Ycoord = Element(3);
Node2ID = Element(4);
Node2Xcoord = Element(5);
Node2Ycoord = Element(6);
MaterialE = Element(7);
Area = Element(8);
Inertia = Element(9);
Nodes = [Node1ID,Node2ID];

% Get distance between nodes
I1 = Node1ID;
I2 = Node2ID;
X21 = Node2Xcoord - Node1Xcoord;
Y21 = Node2Ycoord - Node1Ycoord;
EL = sqrt(X21 * X21 + Y21 * Y21);
EAL = MaterialE * Area / EL;
EIZL = MaterialE * Inertia / EL;
%calculation of density (the uniform load is only taken into account)
SEP = zeros(6);
SEP(1, 1) = EAL;
SEP(1, 4) = -EAL;
SEP(4, 4) = EAL;
SEP(2, 2) = 12 * EIZL / EL ^ 2;
SEP(2, 3) = 6 * EIZL / EL;
SEP(2, 5) = -SEP(2, 2);
SEP(2, 6) = SEP(2, 3);
SEP(3, 3) = 4 * EIZL;
SEP(3, 5) = -6 * EIZL / EL;
SEP(3, 6) = 2 * EIZL;
SEP(5, 5) = 12 * EIZL / EL ^ 2;
SEP(5, 6) = -6 * EIZL / EL;
SEP(6, 6) = 4 * EIZL;
for i = 1:6
   for j = i:6
      SEP(j, i) = SEP(i, j);
   end
end
DCOS = zeros(3,3);
DCOS(1, 1) = X21 / EL;
DCOS(1, 2) = Y21 / EL;
DCOS(1, 3) = 0;
DCOS(2, 1) = -DCOS(1, 2);
DCOS(2, 2) = DCOS(1, 1);
DCOS(2, 3) = 0;
DCOS(3, 1) = 0;
DCOS(3, 2) = 0;
DCOS(3, 3) = 1;
ALMBDA = zeros(6);       
for i = 1:2
   IK = 3 * (i - 1);
   for j = 1:3
      for k = 1:3
         ALMBDA(j + IK, k + IK) = DCOS(j, k);
      end
   end
end
SE = SEP * ALMBDA;
SEP = SE;
SE = ALMBDA' * SEP;
%create the displacement Ue (6x1) vector of the element in global coordinates
Ue = zeros(6,1);
if (I1 * 3) <= NumFreeDOF
    Ue(1, 1) = Displacement(I1 * 3 - 2, 1);
    Ue(2, 1) = Displacement(I1 * 3 - 1, 1);
    Ue(3, 1) = Displacement(I1 * 3, 1);
end
if (I2 * 3) <= NumFreeDOF
    Ue(4, 1) = Displacement(I2 * 3 - 2, 1);
    Ue(5, 1) = Displacement(I2 * 3 - 1, 1);
    Ue(6, 1) = Displacement(I2 * 3, 1);
end
RF = SE * Ue;  %resisting (6x1) resisting force vector of element in global coordinates

== matlab function Generate Element Restoring Forces/Generate Type 1 Element Restoring Force4/Type 1 Element RF ==
  data: Nodes output inherited; Element input inherited; RF output inherited; NumFreeDOF input inherited; Displacement input inherited
% get restoring force for the element
% returns (6x1) restoring force vector of element in global coordinates
function [Nodes,RF] = eml(Element, NumFreeDOF, Displacement)

%% Input mapping
Node1ID = Element(1);
Node1Xcoord = Element(2);
Node1Ycoord = Element(3);
Node2ID = Element(4);
Node2Xcoord = Element(5);
Node2Ycoord = Element(6);
MaterialE = Element(7);
Area = Element(8);
Inertia = Element(9);
Nodes = [Node1ID,Node2ID];

% Get distance between nodes
I1 = Node1ID;
I2 = Node2ID;
X21 = Node2Xcoord - Node1Xcoord;
Y21 = Node2Ycoord - Node1Ycoord;
EL = sqrt(X21 * X21 + Y21 * Y21);
EAL = MaterialE * Area / EL;
EIZL = MaterialE * Inertia / EL;
%calculation of density (the uniform load is only taken into account)
SEP = zeros(6);
SEP(1, 1) = EAL;
SEP(1, 4) = -EAL;
SEP(4, 4) = EAL;
SEP(2, 2) = 12 * EIZL / EL ^ 2;
SEP(2, 3) = 6 * EIZL / EL;
SEP(2, 5) = -SEP(2, 2);
SEP(2, 6) = SEP(2, 3);
SEP(3, 3) = 4 * EIZL;
SEP(3, 5) = -6 * EIZL / EL;
SEP(3, 6) = 2 * EIZL;
SEP(5, 5) = 12 * EIZL / EL ^ 2;
SEP(5, 6) = -6 * EIZL / EL;
SEP(6, 6) = 4 * EIZL;
for i = 1:6
   for j = i:6
      SEP(j, i) = SEP(i, j);
   end
end
DCOS = zeros(3,3);
DCOS(1, 1) = X21 / EL;
DCOS(1, 2) = Y21 / EL;
DCOS(1, 3) = 0;
DCOS(2, 1) = -DCOS(1, 2);
DCOS(2, 2) = DCOS(1, 1);
DCOS(2, 3) = 0;
DCOS(3, 1) = 0;
DCOS(3, 2) = 0;
DCOS(3, 3) = 1;
ALMBDA = zeros(6);       
for i = 1:2
   IK = 3 * (i - 1);
   for j = 1:3
      for k = 1:3
         ALMBDA(j + IK, k + IK) = DCOS(j, k);
      end
   end
end
SE = SEP * ALMBDA;
SEP = SE;
SE = ALMBDA' * SEP;
%create the displacement Ue (6x1) vector of the element in global coordinates
Ue = zeros(6,1);
if (I1 * 3) <= NumFreeDOF
    Ue(1, 1) = Displacement(I1 * 3 - 2, 1);
    Ue(2, 1) = Displacement(I1 * 3 - 1, 1);
    Ue(3, 1) = Displacement(I1 * 3, 1);
end
if (I2 * 3) <= NumFreeDOF
    Ue(4, 1) = Displacement(I2 * 3 - 2, 1);
    Ue(5, 1) = Displacement(I2 * 3 - 1, 1);
    Ue(6, 1) = Displacement(I2 * 3, 1);
end
RF = SE * Ue;  %resisting (6x1) resisting force vector of element in global coordinates

== matlab function Generate Element Restoring Forces/Generate Type 1 Element Restoring Force5/Type 1 Element RF ==
  data: Nodes output inherited; Element input inherited; RF output inherited; NumFreeDOF input inherited; Displacement input inherited
% get restoring force for the element
% returns (6x1) restoring force vector of element in global coordinates
function [Nodes,RF] = eml(Element, NumFreeDOF, Displacement)

%% Input mapping
Node1ID = Element(1);
Node1Xcoord = Element(2);
Node1Ycoord = Element(3);
Node2ID = Element(4);
Node2Xcoord = Element(5);
Node2Ycoord = Element(6);
MaterialE = Element(7);
Area = Element(8);
Inertia = Element(9);
Nodes = [Node1ID,Node2ID];

% Get distance between nodes
I1 = Node1ID;
I2 = Node2ID;
X21 = Node2Xcoord - Node1Xcoord;
Y21 = Node2Ycoord - Node1Ycoord;
EL = sqrt(X21 * X21 + Y21 * Y21);
EAL = MaterialE * Area / EL;
EIZL = MaterialE * Inertia / EL;
%calculation of density (the uniform load is only taken into account)
SEP = zeros(6);
SEP(1, 1) = EAL;
SEP(1, 4) = -EAL;
SEP(4, 4) = EAL;
SEP(2, 2) = 12 * EIZL / EL ^ 2;
SEP(2, 3) = 6 * EIZL / EL;
SEP(2, 5) = -SEP(2, 2);
SEP(2, 6) = SEP(2, 3);
SEP(3, 3) = 4 * EIZL;
SEP(3, 5) = -6 * EIZL / EL;
SEP(3, 6) = 2 * EIZL;
SEP(5, 5) = 12 * EIZL / EL ^ 2;
SEP(5, 6) = -6 * EIZL / EL;
SEP(6, 6) = 4 * EIZL;
for i = 1:6
   for j = i:6
      SEP(j, i) = SEP(i, j);
   end
end
DCOS = zeros(3,3);
DCOS(1, 1) = X21 / EL;
DCOS(1, 2) = Y21 / EL;
DCOS(1, 3) = 0;
DCOS(2, 1) = -DCOS(1, 2);
DCOS(2, 2) = DCOS(1, 1);
DCOS(2, 3) = 0;
DCOS(3, 1) = 0;
DCOS(3, 2) = 0;
DCOS(3, 3) = 1;
ALMBDA = zeros(6);       
for i = 1:2
   IK = 3 * (i - 1);
   for j = 1:3
      for k = 1:3
         ALMBDA(j + IK, k + IK) = DCOS(j, k);
      end
   end
end
SE = SEP * ALMBDA;
SEP = SE;
SE = ALMBDA' * SEP;
%create the displacement Ue (6x1) vector of the element in global coordinates
Ue = zeros(6,1);
if (I1 * 3) <= NumFreeDOF
    Ue(1, 1) = Displacement(I1 * 3 - 2, 1);
    Ue(2, 1) = Displacement(I1 * 3 - 1, 1);
    Ue(3, 1) = Displacement(I1 * 3, 1);
end
if (I2 * 3) <= NumFreeDOF
    Ue(4, 1) = Displacement(I2 * 3 - 2, 1);
    Ue(5, 1) = Displacement(I2 * 3 - 1, 1);
    Ue(6, 1) = Displacement(I2 * 3, 1);
end
RF = SE * Ue;  %resisting (6x1) resisting force vector of element in global coordinates

== matlab function Generate Acceleration Vector/Generate Acceleration Vector ==
  data: TotalRF input inherited; PEFF input inherited; M_FreeInv input inherited; Acceleration output inherited; C_Free input inherited; Velocity input inherited; step_count input inherited
function Acceleration = eml(TotalRF,PEFF,M_FreeInv,C_Free,Velocity,step_count)
% This block supports the Embedded MATLAB subset.
% See the help menu for details. 

Acceleration = M_FreeInv * (PEFF(step_count,:)' - C_Free * Velocity - TotalRF);

== matlab function Generate Command Vectors/Generate Command Vectors ==
  data: Timestep input inherited; Displacement_v output inherited; Beta1 input inherited; Beta2 input inherited; Displacement input inherited; Velocity input inherited; Acceleration input inherited; Velocity_v output inherited
function [Displacement_v,Velocity_v] = eml(Timestep, Beta1, Beta2, Displacement, Velocity, Acceleration)
% This block supports the Embedded MATLAB subset.
% See the help menu for details. 

Displacement_v = Displacement + Timestep*Velocity + Beta2*Timestep^2*Acceleration;
Velocity_v = Velocity + Beta1*Timestep*Acceleration;

== matlab function Generate Element Restoring Forces1/Generate Type 2 Element Restoring Force/Generate Actuator Command ==
  data: Element input inherited; Command output inherited; Displacement input inherited; Velocity input inherited; Timestep input inherited; QuadRampCoeffs output inherited
% get restoring force for the element
% returns (6x1) restoring force vector of element in global coordinates
function [Command, QuadRampCoeffs]  = fcn(Element, Displacement, Velocity, Timestep)

persistent OLD_COMMAND;
persistent COMMAND;
persistent OLD_VELOCITY;
persistent VELOCITY;
if (isempty(OLD_COMMAND))
    OLD_COMMAND = 0;
    COMMAND = 0;
    OLD_VELOCITY = 0;
    VELOCITY = 0;
end

%% Input mapping
Node1ID = Element(1);
Node2ID = Element(2);

% create displacement command
U1 = Displacement(3 * Node1ID - 2, 1);
U2 = Displacement(3 * Node2ID - 2, 1);
OLD_COMMAND = COMMAND;
COMMAND = U2 - U1; 
Command = [COMMAND OLD_COMMAND];

% form local velocity scalar
Ud1 = Velocity(3 * Node1ID - 2, 1);
Ud2 = Velocity(3 * Node2ID - 2, 1);
OLD_VELOCITY = VELOCITY;
VELOCITY = Ud2 - Ud1; 

% Calculate quadratic ramper coefficients
QuadRampCoeffs = zeros(4,1);
QuadRampCoeffs(1) = OLD_COMMAND;
QuadRampCoeffs(2) = OLD_VELOCITY;
QuadRampCoeffs(3) = (-1) * ((Timestep*VELOCITY + 2*OLD_VELOCITY*Timestep + 3*OLD_COMMAND - 3*COMMAND) / Timestep^2);
QuadRampCoeffs(4) = (Timestep*VELOCITY + OLD_VELOCITY*Timestep + 2*OLD_COMMAND - 2*COMMAND) / Timestep^3;
